simulink model "E"  (R2024a)
settings: Solver=VariableStepAuto  StartTime=0.0  StopTime=10*10^-6  RelTol=1e-3
undefined symbols (not defined in the file): c1, c3, rxDpIndex
libraries: commblkcod2 x64, commofdm x64, commdigbbndam3 x64, commsink2 x1, commseqgen3 x1
(part 3 of 3)

== system E/Subsystem1/MCS13 WiFi Demodulator25 ==
  In1 : Inport
  BCH Decoder1 : commblkcod2/BCH Decoder  n=47040  k=39200  specShortening=off  shortenedK=5  specGenPoly=off  genPoly='X^10 + X^8 + X^5 + X^4 + X^2 + X + 1'  specPrimPoly=off  prPoly='X^4 + X + 1'  specDisableGenCheck=off  specPuncture=off  punctVec=[ones(8,1); zeros(2,1)]  specErasurePort=off  showNumErr=off
  OFDM Demodulator1 : commofdm/OFDM Demodulator  StatePerturbationForJacobian=1.0e-05  FFTLength=4096  NumGuardBandCarriers=[88; 88]  RemoveDCCarrier=off  PilotOutputPort=off  PilotCarrierIndices=[35;60;85;110;135;160;185;210;235;260;285;310;335;360;385;410;435;460;485;510;535;560;585;610;635;660;685;710;735;760;785;810;835;860;885;910;935;960;985;1010;1035;1060;1085;1110;1135;1160;1185;1210;1235;1260;1285;1310;1335;1360;1385;1410;1435;1460;1485;1510;1535;1560;1585;1610;1635;1660;1685;1710;1735;1760;1785;1810;1835;1860;1885;1910;1935;1960;1985;2010;2035]  CyclicPrefixLength=0  OversamplingFactor=1  NumSymbols=1  NumReceiveAntennas=1  SimulateUsing=Interpreted execution
  Rectangular QAM Demodulator Baseband1 : commdigbbndam3/Rectangular QAM Demodulator Baseband  M=4096  OutType=Bit  DecType=Hard decision  VarSource=Dialog  Variance=1  Dec=Gray  Mapping=[0:15]  PowType=Min. distance between symbols  MinDist=2  AvgPow=1  PeakPow=1  Ph=0  outDtype1=Inherit via internal rule  outDtype2=Inherit via internal rule  derotateFactorWordLen=16  derotateFactorDataTypeStr=Inherit: Same word length as input  derotateFactorLastDataTypeStr=Inherit: Same word length as input  denormFactorWordLen=16  denormFactorDataTypeStr=Inherit: Same word length as input  denormFactorLastDataTypeStr=Inherit: Same word length as input  prodOutWordLen=32  prodOutOverflowMode=Wrap  prodOutRoundingMode=Floor  prodOutOvFlMode=off  prodOutOvFlModeLastStrValue=off  sumWordLen=32
      settings: LibrarySourceBlock=|
      | commhdldigbbndam/Rectangular QAM
      | Demodulator
      | Baseband
  Out1 : Outport
  wires:
  BCH Decoder1/1 -> Out1/1
  OFDM Demodulator1/1 -> Rectangular QAM Demodulator Baseband1/1
  In1/1 -> OFDM Demodulator1/1
  Rectangular QAM Demodulator Baseband1/1 -> BCH Decoder1/1

== system E/Subsystem1/MCS13 WiFi Demodulator26 ==
  In1 : Inport
  BCH Decoder1 : commblkcod2/BCH Decoder  n=47040  k=39200  specShortening=off  shortenedK=5  specGenPoly=off  genPoly='X^10 + X^8 + X^5 + X^4 + X^2 + X + 1'  specPrimPoly=off  prPoly='X^4 + X + 1'  specDisableGenCheck=off  specPuncture=off  punctVec=[ones(8,1); zeros(2,1)]  specErasurePort=off  showNumErr=off
  OFDM Demodulator1 : commofdm/OFDM Demodulator  StatePerturbationForJacobian=1.0e-05  FFTLength=4096  NumGuardBandCarriers=[88; 88]  RemoveDCCarrier=off  PilotOutputPort=off  PilotCarrierIndices=[35;60;85;110;135;160;185;210;235;260;285;310;335;360;385;410;435;460;485;510;535;560;585;610;635;660;685;710;735;760;785;810;835;860;885;910;935;960;985;1010;1035;1060;1085;1110;1135;1160;1185;1210;1235;1260;1285;1310;1335;1360;1385;1410;1435;1460;1485;1510;1535;1560;1585;1610;1635;1660;1685;1710;1735;1760;1785;1810;1835;1860;1885;1910;1935;1960;1985;2010;2035]  CyclicPrefixLength=0  OversamplingFactor=1  NumSymbols=1  NumReceiveAntennas=1  SimulateUsing=Interpreted execution
  Rectangular QAM Demodulator Baseband1 : commdigbbndam3/Rectangular QAM Demodulator Baseband  M=4096  OutType=Bit  DecType=Hard decision  VarSource=Dialog  Variance=1  Dec=Gray  Mapping=[0:15]  PowType=Min. distance between symbols  MinDist=2  AvgPow=1  PeakPow=1  Ph=0  outDtype1=Inherit via internal rule  outDtype2=Inherit via internal rule  derotateFactorWordLen=16  derotateFactorDataTypeStr=Inherit: Same word length as input  derotateFactorLastDataTypeStr=Inherit: Same word length as input  denormFactorWordLen=16  denormFactorDataTypeStr=Inherit: Same word length as input  denormFactorLastDataTypeStr=Inherit: Same word length as input  prodOutWordLen=32  prodOutOverflowMode=Wrap  prodOutRoundingMode=Floor  prodOutOvFlMode=off  prodOutOvFlModeLastStrValue=off  sumWordLen=32
      settings: LibrarySourceBlock=|
      | commhdldigbbndam/Rectangular QAM
      | Demodulator
      | Baseband
  Out1 : Outport
  wires:
  BCH Decoder1/1 -> Out1/1
  OFDM Demodulator1/1 -> Rectangular QAM Demodulator Baseband1/1
  In1/1 -> OFDM Demodulator1/1
  Rectangular QAM Demodulator Baseband1/1 -> BCH Decoder1/1

== system E/Subsystem1/MCS13 WiFi Demodulator27 ==
  In1 : Inport
  BCH Decoder1 : commblkcod2/BCH Decoder  n=47040  k=39200  specShortening=off  shortenedK=5  specGenPoly=off  genPoly='X^10 + X^8 + X^5 + X^4 + X^2 + X + 1'  specPrimPoly=off  prPoly='X^4 + X + 1'  specDisableGenCheck=off  specPuncture=off  punctVec=[ones(8,1); zeros(2,1)]  specErasurePort=off  showNumErr=off
  OFDM Demodulator1 : commofdm/OFDM Demodulator  StatePerturbationForJacobian=1.0e-05  FFTLength=4096  NumGuardBandCarriers=[88; 88]  RemoveDCCarrier=off  PilotOutputPort=off  PilotCarrierIndices=[35;60;85;110;135;160;185;210;235;260;285;310;335;360;385;410;435;460;485;510;535;560;585;610;635;660;685;710;735;760;785;810;835;860;885;910;935;960;985;1010;1035;1060;1085;1110;1135;1160;1185;1210;1235;1260;1285;1310;1335;1360;1385;1410;1435;1460;1485;1510;1535;1560;1585;1610;1635;1660;1685;1710;1735;1760;1785;1810;1835;1860;1885;1910;1935;1960;1985;2010;2035]  CyclicPrefixLength=0  OversamplingFactor=1  NumSymbols=1  NumReceiveAntennas=1  SimulateUsing=Interpreted execution
  Rectangular QAM Demodulator Baseband1 : commdigbbndam3/Rectangular QAM Demodulator Baseband  M=4096  OutType=Bit  DecType=Hard decision  VarSource=Dialog  Variance=1  Dec=Gray  Mapping=[0:15]  PowType=Min. distance between symbols  MinDist=2  AvgPow=1  PeakPow=1  Ph=0  outDtype1=Inherit via internal rule  outDtype2=Inherit via internal rule  derotateFactorWordLen=16  derotateFactorDataTypeStr=Inherit: Same word length as input  derotateFactorLastDataTypeStr=Inherit: Same word length as input  denormFactorWordLen=16  denormFactorDataTypeStr=Inherit: Same word length as input  denormFactorLastDataTypeStr=Inherit: Same word length as input  prodOutWordLen=32  prodOutOverflowMode=Wrap  prodOutRoundingMode=Floor  prodOutOvFlMode=off  prodOutOvFlModeLastStrValue=off  sumWordLen=32
      settings: LibrarySourceBlock=|
      | commhdldigbbndam/Rectangular QAM
      | Demodulator
      | Baseband
  Out1 : Outport
  wires:
  BCH Decoder1/1 -> Out1/1
  OFDM Demodulator1/1 -> Rectangular QAM Demodulator Baseband1/1
  In1/1 -> OFDM Demodulator1/1
  Rectangular QAM Demodulator Baseband1/1 -> BCH Decoder1/1

== system E/Subsystem1/MCS13 WiFi Demodulator28 ==
  In1 : Inport
  BCH Decoder1 : commblkcod2/BCH Decoder  n=47040  k=39200  specShortening=off  shortenedK=5  specGenPoly=off  genPoly='X^10 + X^8 + X^5 + X^4 + X^2 + X + 1'  specPrimPoly=off  prPoly='X^4 + X + 1'  specDisableGenCheck=off  specPuncture=off  punctVec=[ones(8,1); zeros(2,1)]  specErasurePort=off  showNumErr=off
  OFDM Demodulator1 : commofdm/OFDM Demodulator  StatePerturbationForJacobian=1.0e-05  FFTLength=4096  NumGuardBandCarriers=[88; 88]  RemoveDCCarrier=off  PilotOutputPort=off  PilotCarrierIndices=[35;60;85;110;135;160;185;210;235;260;285;310;335;360;385;410;435;460;485;510;535;560;585;610;635;660;685;710;735;760;785;810;835;860;885;910;935;960;985;1010;1035;1060;1085;1110;1135;1160;1185;1210;1235;1260;1285;1310;1335;1360;1385;1410;1435;1460;1485;1510;1535;1560;1585;1610;1635;1660;1685;1710;1735;1760;1785;1810;1835;1860;1885;1910;1935;1960;1985;2010;2035]  CyclicPrefixLength=0  OversamplingFactor=1  NumSymbols=1  NumReceiveAntennas=1  SimulateUsing=Interpreted execution
  Rectangular QAM Demodulator Baseband1 : commdigbbndam3/Rectangular QAM Demodulator Baseband  M=4096  OutType=Bit  DecType=Hard decision  VarSource=Dialog  Variance=1  Dec=Gray  Mapping=[0:15]  PowType=Min. distance between symbols  MinDist=2  AvgPow=1  PeakPow=1  Ph=0  outDtype1=Inherit via internal rule  outDtype2=Inherit via internal rule  derotateFactorWordLen=16  derotateFactorDataTypeStr=Inherit: Same word length as input  derotateFactorLastDataTypeStr=Inherit: Same word length as input  denormFactorWordLen=16  denormFactorDataTypeStr=Inherit: Same word length as input  denormFactorLastDataTypeStr=Inherit: Same word length as input  prodOutWordLen=32  prodOutOverflowMode=Wrap  prodOutRoundingMode=Floor  prodOutOvFlMode=off  prodOutOvFlModeLastStrValue=off  sumWordLen=32
      settings: LibrarySourceBlock=|
      | commhdldigbbndam/Rectangular QAM
      | Demodulator
      | Baseband
  Out1 : Outport
  wires:
  BCH Decoder1/1 -> Out1/1
  OFDM Demodulator1/1 -> Rectangular QAM Demodulator Baseband1/1
  In1/1 -> OFDM Demodulator1/1
  Rectangular QAM Demodulator Baseband1/1 -> BCH Decoder1/1

== system E/Subsystem1/MCS13 WiFi Demodulator29 ==
  In1 : Inport
  BCH Decoder1 : commblkcod2/BCH Decoder  n=47040  k=39200  specShortening=off  shortenedK=5  specGenPoly=off  genPoly='X^10 + X^8 + X^5 + X^4 + X^2 + X + 1'  specPrimPoly=off  prPoly='X^4 + X + 1'  specDisableGenCheck=off  specPuncture=off  punctVec=[ones(8,1); zeros(2,1)]  specErasurePort=off  showNumErr=off
  OFDM Demodulator1 : commofdm/OFDM Demodulator  StatePerturbationForJacobian=1.0e-05  FFTLength=4096  NumGuardBandCarriers=[88; 88]  RemoveDCCarrier=off  PilotOutputPort=off  PilotCarrierIndices=[35;60;85;110;135;160;185;210;235;260;285;310;335;360;385;410;435;460;485;510;535;560;585;610;635;660;685;710;735;760;785;810;835;860;885;910;935;960;985;1010;1035;1060;1085;1110;1135;1160;1185;1210;1235;1260;1285;1310;1335;1360;1385;1410;1435;1460;1485;1510;1535;1560;1585;1610;1635;1660;1685;1710;1735;1760;1785;1810;1835;1860;1885;1910;1935;1960;1985;2010;2035]  CyclicPrefixLength=0  OversamplingFactor=1  NumSymbols=1  NumReceiveAntennas=1  SimulateUsing=Interpreted execution
  Rectangular QAM Demodulator Baseband1 : commdigbbndam3/Rectangular QAM Demodulator Baseband  M=4096  OutType=Bit  DecType=Hard decision  VarSource=Dialog  Variance=1  Dec=Gray  Mapping=[0:15]  PowType=Min. distance between symbols  MinDist=2  AvgPow=1  PeakPow=1  Ph=0  outDtype1=Inherit via internal rule  outDtype2=Inherit via internal rule  derotateFactorWordLen=16  derotateFactorDataTypeStr=Inherit: Same word length as input  derotateFactorLastDataTypeStr=Inherit: Same word length as input  denormFactorWordLen=16  denormFactorDataTypeStr=Inherit: Same word length as input  denormFactorLastDataTypeStr=Inherit: Same word length as input  prodOutWordLen=32  prodOutOverflowMode=Wrap  prodOutRoundingMode=Floor  prodOutOvFlMode=off  prodOutOvFlModeLastStrValue=off  sumWordLen=32
      settings: LibrarySourceBlock=|
      | commhdldigbbndam/Rectangular QAM
      | Demodulator
      | Baseband
  Out1 : Outport
  wires:
  BCH Decoder1/1 -> Out1/1
  OFDM Demodulator1/1 -> Rectangular QAM Demodulator Baseband1/1
  In1/1 -> OFDM Demodulator1/1
  Rectangular QAM Demodulator Baseband1/1 -> BCH Decoder1/1

== system E/Subsystem1/MCS13 WiFi Demodulator3 ==
  In1 : Inport
  BCH Decoder1 : commblkcod2/BCH Decoder  n=47040  k=39200  specShortening=off  shortenedK=5  specGenPoly=off  genPoly='X^10 + X^8 + X^5 + X^4 + X^2 + X + 1'  specPrimPoly=off  prPoly='X^4 + X + 1'  specDisableGenCheck=off  specPuncture=off  punctVec=[ones(8,1); zeros(2,1)]  specErasurePort=off  showNumErr=off
  OFDM Demodulator1 : commofdm/OFDM Demodulator  StatePerturbationForJacobian=1.0e-05  FFTLength=4096  NumGuardBandCarriers=[88; 88]  RemoveDCCarrier=off  PilotOutputPort=off  PilotCarrierIndices=[35;60;85;110;135;160;185;210;235;260;285;310;335;360;385;410;435;460;485;510;535;560;585;610;635;660;685;710;735;760;785;810;835;860;885;910;935;960;985;1010;1035;1060;1085;1110;1135;1160;1185;1210;1235;1260;1285;1310;1335;1360;1385;1410;1435;1460;1485;1510;1535;1560;1585;1610;1635;1660;1685;1710;1735;1760;1785;1810;1835;1860;1885;1910;1935;1960;1985;2010;2035]  CyclicPrefixLength=0  OversamplingFactor=1  NumSymbols=1  NumReceiveAntennas=1  SimulateUsing=Interpreted execution
  Rectangular QAM Demodulator Baseband1 : commdigbbndam3/Rectangular QAM Demodulator Baseband  M=4096  OutType=Bit  DecType=Hard decision  VarSource=Dialog  Variance=1  Dec=Gray  Mapping=[0:15]  PowType=Min. distance between symbols  MinDist=2  AvgPow=1  PeakPow=1  Ph=0  outDtype1=Inherit via internal rule  outDtype2=Inherit via internal rule  derotateFactorWordLen=16  derotateFactorDataTypeStr=Inherit: Same word length as input  derotateFactorLastDataTypeStr=Inherit: Same word length as input  denormFactorWordLen=16  denormFactorDataTypeStr=Inherit: Same word length as input  denormFactorLastDataTypeStr=Inherit: Same word length as input  prodOutWordLen=32  prodOutOverflowMode=Wrap  prodOutRoundingMode=Floor  prodOutOvFlMode=off  prodOutOvFlModeLastStrValue=off  sumWordLen=32
      settings: LibrarySourceBlock=|
      | commhdldigbbndam/Rectangular QAM
      | Demodulator
      | Baseband
  Out1 : Outport
  wires:
  BCH Decoder1/1 -> Out1/1
  OFDM Demodulator1/1 -> Rectangular QAM Demodulator Baseband1/1
  In1/1 -> OFDM Demodulator1/1
  Rectangular QAM Demodulator Baseband1/1 -> BCH Decoder1/1

== system E/Subsystem1/MCS13 WiFi Demodulator30 ==
  In1 : Inport
  BCH Decoder1 : commblkcod2/BCH Decoder  n=47040  k=39200  specShortening=off  shortenedK=5  specGenPoly=off  genPoly='X^10 + X^8 + X^5 + X^4 + X^2 + X + 1'  specPrimPoly=off  prPoly='X^4 + X + 1'  specDisableGenCheck=off  specPuncture=off  punctVec=[ones(8,1); zeros(2,1)]  specErasurePort=off  showNumErr=off
  OFDM Demodulator1 : commofdm/OFDM Demodulator  StatePerturbationForJacobian=1.0e-05  FFTLength=4096  NumGuardBandCarriers=[88; 88]  RemoveDCCarrier=off  PilotOutputPort=off  PilotCarrierIndices=[35;60;85;110;135;160;185;210;235;260;285;310;335;360;385;410;435;460;485;510;535;560;585;610;635;660;685;710;735;760;785;810;835;860;885;910;935;960;985;1010;1035;1060;1085;1110;1135;1160;1185;1210;1235;1260;1285;1310;1335;1360;1385;1410;1435;1460;1485;1510;1535;1560;1585;1610;1635;1660;1685;1710;1735;1760;1785;1810;1835;1860;1885;1910;1935;1960;1985;2010;2035]  CyclicPrefixLength=0  OversamplingFactor=1  NumSymbols=1  NumReceiveAntennas=1  SimulateUsing=Interpreted execution
  Rectangular QAM Demodulator Baseband1 : commdigbbndam3/Rectangular QAM Demodulator Baseband  M=4096  OutType=Bit  DecType=Hard decision  VarSource=Dialog  Variance=1  Dec=Gray  Mapping=[0:15]  PowType=Min. distance between symbols  MinDist=2  AvgPow=1  PeakPow=1  Ph=0  outDtype1=Inherit via internal rule  outDtype2=Inherit via internal rule  derotateFactorWordLen=16  derotateFactorDataTypeStr=Inherit: Same word length as input  derotateFactorLastDataTypeStr=Inherit: Same word length as input  denormFactorWordLen=16  denormFactorDataTypeStr=Inherit: Same word length as input  denormFactorLastDataTypeStr=Inherit: Same word length as input  prodOutWordLen=32  prodOutOverflowMode=Wrap  prodOutRoundingMode=Floor  prodOutOvFlMode=off  prodOutOvFlModeLastStrValue=off  sumWordLen=32
      settings: LibrarySourceBlock=|
      | commhdldigbbndam/Rectangular QAM
      | Demodulator
      | Baseband
  Out1 : Outport
  wires:
  BCH Decoder1/1 -> Out1/1
  OFDM Demodulator1/1 -> Rectangular QAM Demodulator Baseband1/1
  In1/1 -> OFDM Demodulator1/1
  Rectangular QAM Demodulator Baseband1/1 -> BCH Decoder1/1

== system E/Subsystem1/MCS13 WiFi Demodulator31 ==
  In1 : Inport
  BCH Decoder1 : commblkcod2/BCH Decoder  n=47040  k=39200  specShortening=off  shortenedK=5  specGenPoly=off  genPoly='X^10 + X^8 + X^5 + X^4 + X^2 + X + 1'  specPrimPoly=off  prPoly='X^4 + X + 1'  specDisableGenCheck=off  specPuncture=off  punctVec=[ones(8,1); zeros(2,1)]  specErasurePort=off  showNumErr=off
  OFDM Demodulator1 : commofdm/OFDM Demodulator  StatePerturbationForJacobian=1.0e-05  FFTLength=4096  NumGuardBandCarriers=[88; 88]  RemoveDCCarrier=off  PilotOutputPort=off  PilotCarrierIndices=[35;60;85;110;135;160;185;210;235;260;285;310;335;360;385;410;435;460;485;510;535;560;585;610;635;660;685;710;735;760;785;810;835;860;885;910;935;960;985;1010;1035;1060;1085;1110;1135;1160;1185;1210;1235;1260;1285;1310;1335;1360;1385;1410;1435;1460;1485;1510;1535;1560;1585;1610;1635;1660;1685;1710;1735;1760;1785;1810;1835;1860;1885;1910;1935;1960;1985;2010;2035]  CyclicPrefixLength=0  OversamplingFactor=1  NumSymbols=1  NumReceiveAntennas=1  SimulateUsing=Interpreted execution
  Rectangular QAM Demodulator Baseband1 : commdigbbndam3/Rectangular QAM Demodulator Baseband  M=4096  OutType=Bit  DecType=Hard decision  VarSource=Dialog  Variance=1  Dec=Gray  Mapping=[0:15]  PowType=Min. distance between symbols  MinDist=2  AvgPow=1  PeakPow=1  Ph=0  outDtype1=Inherit via internal rule  outDtype2=Inherit via internal rule  derotateFactorWordLen=16  derotateFactorDataTypeStr=Inherit: Same word length as input  derotateFactorLastDataTypeStr=Inherit: Same word length as input  denormFactorWordLen=16  denormFactorDataTypeStr=Inherit: Same word length as input  denormFactorLastDataTypeStr=Inherit: Same word length as input  prodOutWordLen=32  prodOutOverflowMode=Wrap  prodOutRoundingMode=Floor  prodOutOvFlMode=off  prodOutOvFlModeLastStrValue=off  sumWordLen=32
      settings: LibrarySourceBlock=|
      | commhdldigbbndam/Rectangular QAM
      | Demodulator
      | Baseband
  Out1 : Outport
  wires:
  BCH Decoder1/1 -> Out1/1
  OFDM Demodulator1/1 -> Rectangular QAM Demodulator Baseband1/1
  In1/1 -> OFDM Demodulator1/1
  Rectangular QAM Demodulator Baseband1/1 -> BCH Decoder1/1

== system E/Subsystem1/MCS13 WiFi Demodulator32 ==
  In1 : Inport
  BCH Decoder1 : commblkcod2/BCH Decoder  n=47040  k=39200  specShortening=off  shortenedK=5  specGenPoly=off  genPoly='X^10 + X^8 + X^5 + X^4 + X^2 + X + 1'  specPrimPoly=off  prPoly='X^4 + X + 1'  specDisableGenCheck=off  specPuncture=off  punctVec=[ones(8,1); zeros(2,1)]  specErasurePort=off  showNumErr=off
  OFDM Demodulator1 : commofdm/OFDM Demodulator  StatePerturbationForJacobian=1.0e-05  FFTLength=4096  NumGuardBandCarriers=[88; 88]  RemoveDCCarrier=off  PilotOutputPort=off  PilotCarrierIndices=[35;60;85;110;135;160;185;210;235;260;285;310;335;360;385;410;435;460;485;510;535;560;585;610;635;660;685;710;735;760;785;810;835;860;885;910;935;960;985;1010;1035;1060;1085;1110;1135;1160;1185;1210;1235;1260;1285;1310;1335;1360;1385;1410;1435;1460;1485;1510;1535;1560;1585;1610;1635;1660;1685;1710;1735;1760;1785;1810;1835;1860;1885;1910;1935;1960;1985;2010;2035]  CyclicPrefixLength=0  OversamplingFactor=1  NumSymbols=1  NumReceiveAntennas=1  SimulateUsing=Interpreted execution
  Rectangular QAM Demodulator Baseband1 : commdigbbndam3/Rectangular QAM Demodulator Baseband  M=4096  OutType=Bit  DecType=Hard decision  VarSource=Dialog  Variance=1  Dec=Gray  Mapping=[0:15]  PowType=Min. distance between symbols  MinDist=2  AvgPow=1  PeakPow=1  Ph=0  outDtype1=Inherit via internal rule  outDtype2=Inherit via internal rule  derotateFactorWordLen=16  derotateFactorDataTypeStr=Inherit: Same word length as input  derotateFactorLastDataTypeStr=Inherit: Same word length as input  denormFactorWordLen=16  denormFactorDataTypeStr=Inherit: Same word length as input  denormFactorLastDataTypeStr=Inherit: Same word length as input  prodOutWordLen=32  prodOutOverflowMode=Wrap  prodOutRoundingMode=Floor  prodOutOvFlMode=off  prodOutOvFlModeLastStrValue=off  sumWordLen=32
      settings: LibrarySourceBlock=|
      | commhdldigbbndam/Rectangular QAM
      | Demodulator
      | Baseband
  Out1 : Outport
  wires:
  BCH Decoder1/1 -> Out1/1
  OFDM Demodulator1/1 -> Rectangular QAM Demodulator Baseband1/1
  In1/1 -> OFDM Demodulator1/1
  Rectangular QAM Demodulator Baseband1/1 -> BCH Decoder1/1

== system E/Subsystem1/MCS13 WiFi Demodulator4 ==
  In1 : Inport
  BCH Decoder1 : commblkcod2/BCH Decoder  n=47040  k=39200  specShortening=off  shortenedK=5  specGenPoly=off  genPoly='X^10 + X^8 + X^5 + X^4 + X^2 + X + 1'  specPrimPoly=off  prPoly='X^4 + X + 1'  specDisableGenCheck=off  specPuncture=off  punctVec=[ones(8,1); zeros(2,1)]  specErasurePort=off  showNumErr=off
  OFDM Demodulator1 : commofdm/OFDM Demodulator  StatePerturbationForJacobian=1.0e-05  FFTLength=4096  NumGuardBandCarriers=[88; 88]  RemoveDCCarrier=off  PilotOutputPort=off  PilotCarrierIndices=[35;60;85;110;135;160;185;210;235;260;285;310;335;360;385;410;435;460;485;510;535;560;585;610;635;660;685;710;735;760;785;810;835;860;885;910;935;960;985;1010;1035;1060;1085;1110;1135;1160;1185;1210;1235;1260;1285;1310;1335;1360;1385;1410;1435;1460;1485;1510;1535;1560;1585;1610;1635;1660;1685;1710;1735;1760;1785;1810;1835;1860;1885;1910;1935;1960;1985;2010;2035]  CyclicPrefixLength=0  OversamplingFactor=1  NumSymbols=1  NumReceiveAntennas=1  SimulateUsing=Interpreted execution
  Rectangular QAM Demodulator Baseband1 : commdigbbndam3/Rectangular QAM Demodulator Baseband  M=4096  OutType=Bit  DecType=Hard decision  VarSource=Dialog  Variance=1  Dec=Gray  Mapping=[0:15]  PowType=Min. distance between symbols  MinDist=2  AvgPow=1  PeakPow=1  Ph=0  outDtype1=Inherit via internal rule  outDtype2=Inherit via internal rule  derotateFactorWordLen=16  derotateFactorDataTypeStr=Inherit: Same word length as input  derotateFactorLastDataTypeStr=Inherit: Same word length as input  denormFactorWordLen=16  denormFactorDataTypeStr=Inherit: Same word length as input  denormFactorLastDataTypeStr=Inherit: Same word length as input  prodOutWordLen=32  prodOutOverflowMode=Wrap  prodOutRoundingMode=Floor  prodOutOvFlMode=off  prodOutOvFlModeLastStrValue=off  sumWordLen=32
      settings: LibrarySourceBlock=|
      | commhdldigbbndam/Rectangular QAM
      | Demodulator
      | Baseband
  Out1 : Outport
  wires:
  BCH Decoder1/1 -> Out1/1
  OFDM Demodulator1/1 -> Rectangular QAM Demodulator Baseband1/1
  In1/1 -> OFDM Demodulator1/1
  Rectangular QAM Demodulator Baseband1/1 -> BCH Decoder1/1

== system E/Subsystem1/MCS13 WiFi Demodulator5 ==
  In1 : Inport
  BCH Decoder1 : commblkcod2/BCH Decoder  n=47040  k=39200  specShortening=off  shortenedK=5  specGenPoly=off  genPoly='X^10 + X^8 + X^5 + X^4 + X^2 + X + 1'  specPrimPoly=off  prPoly='X^4 + X + 1'  specDisableGenCheck=off  specPuncture=off  punctVec=[ones(8,1); zeros(2,1)]  specErasurePort=off  showNumErr=off
  OFDM Demodulator1 : commofdm/OFDM Demodulator  StatePerturbationForJacobian=1.0e-05  FFTLength=4096  NumGuardBandCarriers=[88; 88]  RemoveDCCarrier=off  PilotOutputPort=off  PilotCarrierIndices=[35;60;85;110;135;160;185;210;235;260;285;310;335;360;385;410;435;460;485;510;535;560;585;610;635;660;685;710;735;760;785;810;835;860;885;910;935;960;985;1010;1035;1060;1085;1110;1135;1160;1185;1210;1235;1260;1285;1310;1335;1360;1385;1410;1435;1460;1485;1510;1535;1560;1585;1610;1635;1660;1685;1710;1735;1760;1785;1810;1835;1860;1885;1910;1935;1960;1985;2010;2035]  CyclicPrefixLength=0  OversamplingFactor=1  NumSymbols=1  NumReceiveAntennas=1  SimulateUsing=Interpreted execution
  Rectangular QAM Demodulator Baseband1 : commdigbbndam3/Rectangular QAM Demodulator Baseband  M=4096  OutType=Bit  DecType=Hard decision  VarSource=Dialog  Variance=1  Dec=Gray  Mapping=[0:15]  PowType=Min. distance between symbols  MinDist=2  AvgPow=1  PeakPow=1  Ph=0  outDtype1=Inherit via internal rule  outDtype2=Inherit via internal rule  derotateFactorWordLen=16  derotateFactorDataTypeStr=Inherit: Same word length as input  derotateFactorLastDataTypeStr=Inherit: Same word length as input  denormFactorWordLen=16  denormFactorDataTypeStr=Inherit: Same word length as input  denormFactorLastDataTypeStr=Inherit: Same word length as input  prodOutWordLen=32  prodOutOverflowMode=Wrap  prodOutRoundingMode=Floor  prodOutOvFlMode=off  prodOutOvFlModeLastStrValue=off  sumWordLen=32
      settings: LibrarySourceBlock=|
      | commhdldigbbndam/Rectangular QAM
      | Demodulator
      | Baseband
  Out1 : Outport
  wires:
  BCH Decoder1/1 -> Out1/1
  OFDM Demodulator1/1 -> Rectangular QAM Demodulator Baseband1/1
  In1/1 -> OFDM Demodulator1/1
  Rectangular QAM Demodulator Baseband1/1 -> BCH Decoder1/1

== system E/Subsystem1/MCS13 WiFi Demodulator6 ==
  In1 : Inport
  BCH Decoder1 : commblkcod2/BCH Decoder  n=47040  k=39200  specShortening=off  shortenedK=5  specGenPoly=off  genPoly='X^10 + X^8 + X^5 + X^4 + X^2 + X + 1'  specPrimPoly=off  prPoly='X^4 + X + 1'  specDisableGenCheck=off  specPuncture=off  punctVec=[ones(8,1); zeros(2,1)]  specErasurePort=off  showNumErr=off
  OFDM Demodulator1 : commofdm/OFDM Demodulator  StatePerturbationForJacobian=1.0e-05  FFTLength=4096  NumGuardBandCarriers=[88; 88]  RemoveDCCarrier=off  PilotOutputPort=off  PilotCarrierIndices=[35;60;85;110;135;160;185;210;235;260;285;310;335;360;385;410;435;460;485;510;535;560;585;610;635;660;685;710;735;760;785;810;835;860;885;910;935;960;985;1010;1035;1060;1085;1110;1135;1160;1185;1210;1235;1260;1285;1310;1335;1360;1385;1410;1435;1460;1485;1510;1535;1560;1585;1610;1635;1660;1685;1710;1735;1760;1785;1810;1835;1860;1885;1910;1935;1960;1985;2010;2035]  CyclicPrefixLength=0  OversamplingFactor=1  NumSymbols=1  NumReceiveAntennas=1  SimulateUsing=Interpreted execution
  Rectangular QAM Demodulator Baseband1 : commdigbbndam3/Rectangular QAM Demodulator Baseband  M=4096  OutType=Bit  DecType=Hard decision  VarSource=Dialog  Variance=1  Dec=Gray  Mapping=[0:15]  PowType=Min. distance between symbols  MinDist=2  AvgPow=1  PeakPow=1  Ph=0  outDtype1=Inherit via internal rule  outDtype2=Inherit via internal rule  derotateFactorWordLen=16  derotateFactorDataTypeStr=Inherit: Same word length as input  derotateFactorLastDataTypeStr=Inherit: Same word length as input  denormFactorWordLen=16  denormFactorDataTypeStr=Inherit: Same word length as input  denormFactorLastDataTypeStr=Inherit: Same word length as input  prodOutWordLen=32  prodOutOverflowMode=Wrap  prodOutRoundingMode=Floor  prodOutOvFlMode=off  prodOutOvFlModeLastStrValue=off  sumWordLen=32
      settings: LibrarySourceBlock=|
      | commhdldigbbndam/Rectangular QAM
      | Demodulator
      | Baseband
  Out1 : Outport
  wires:
  BCH Decoder1/1 -> Out1/1
  OFDM Demodulator1/1 -> Rectangular QAM Demodulator Baseband1/1
  In1/1 -> OFDM Demodulator1/1
  Rectangular QAM Demodulator Baseband1/1 -> BCH Decoder1/1

== system E/Subsystem1/MCS13 WiFi Demodulator7 ==
  In1 : Inport
  BCH Decoder1 : commblkcod2/BCH Decoder  n=47040  k=39200  specShortening=off  shortenedK=5  specGenPoly=off  genPoly='X^10 + X^8 + X^5 + X^4 + X^2 + X + 1'  specPrimPoly=off  prPoly='X^4 + X + 1'  specDisableGenCheck=off  specPuncture=off  punctVec=[ones(8,1); zeros(2,1)]  specErasurePort=off  showNumErr=off
  OFDM Demodulator1 : commofdm/OFDM Demodulator  StatePerturbationForJacobian=1.0e-05  FFTLength=4096  NumGuardBandCarriers=[88; 88]  RemoveDCCarrier=off  PilotOutputPort=off  PilotCarrierIndices=[35;60;85;110;135;160;185;210;235;260;285;310;335;360;385;410;435;460;485;510;535;560;585;610;635;660;685;710;735;760;785;810;835;860;885;910;935;960;985;1010;1035;1060;1085;1110;1135;1160;1185;1210;1235;1260;1285;1310;1335;1360;1385;1410;1435;1460;1485;1510;1535;1560;1585;1610;1635;1660;1685;1710;1735;1760;1785;1810;1835;1860;1885;1910;1935;1960;1985;2010;2035]  CyclicPrefixLength=0  OversamplingFactor=1  NumSymbols=1  NumReceiveAntennas=1  SimulateUsing=Interpreted execution
  Rectangular QAM Demodulator Baseband1 : commdigbbndam3/Rectangular QAM Demodulator Baseband  M=4096  OutType=Bit  DecType=Hard decision  VarSource=Dialog  Variance=1  Dec=Gray  Mapping=[0:15]  PowType=Min. distance between symbols  MinDist=2  AvgPow=1  PeakPow=1  Ph=0  outDtype1=Inherit via internal rule  outDtype2=Inherit via internal rule  derotateFactorWordLen=16  derotateFactorDataTypeStr=Inherit: Same word length as input  derotateFactorLastDataTypeStr=Inherit: Same word length as input  denormFactorWordLen=16  denormFactorDataTypeStr=Inherit: Same word length as input  denormFactorLastDataTypeStr=Inherit: Same word length as input  prodOutWordLen=32  prodOutOverflowMode=Wrap  prodOutRoundingMode=Floor  prodOutOvFlMode=off  prodOutOvFlModeLastStrValue=off  sumWordLen=32
      settings: LibrarySourceBlock=|
      | commhdldigbbndam/Rectangular QAM
      | Demodulator
      | Baseband
  Out1 : Outport
  wires:
  BCH Decoder1/1 -> Out1/1
  OFDM Demodulator1/1 -> Rectangular QAM Demodulator Baseband1/1
  In1/1 -> OFDM Demodulator1/1
  Rectangular QAM Demodulator Baseband1/1 -> BCH Decoder1/1

== system E/Subsystem1/MCS13 WiFi Demodulator8 ==
  In1 : Inport
  BCH Decoder1 : commblkcod2/BCH Decoder  n=47040  k=39200  specShortening=off  shortenedK=5  specGenPoly=off  genPoly='X^10 + X^8 + X^5 + X^4 + X^2 + X + 1'  specPrimPoly=off  prPoly='X^4 + X + 1'  specDisableGenCheck=off  specPuncture=off  punctVec=[ones(8,1); zeros(2,1)]  specErasurePort=off  showNumErr=off
  OFDM Demodulator1 : commofdm/OFDM Demodulator  StatePerturbationForJacobian=1.0e-05  FFTLength=4096  NumGuardBandCarriers=[88; 88]  RemoveDCCarrier=off  PilotOutputPort=off  PilotCarrierIndices=[35;60;85;110;135;160;185;210;235;260;285;310;335;360;385;410;435;460;485;510;535;560;585;610;635;660;685;710;735;760;785;810;835;860;885;910;935;960;985;1010;1035;1060;1085;1110;1135;1160;1185;1210;1235;1260;1285;1310;1335;1360;1385;1410;1435;1460;1485;1510;1535;1560;1585;1610;1635;1660;1685;1710;1735;1760;1785;1810;1835;1860;1885;1910;1935;1960;1985;2010;2035]  CyclicPrefixLength=0  OversamplingFactor=1  NumSymbols=1  NumReceiveAntennas=1  SimulateUsing=Interpreted execution
  Rectangular QAM Demodulator Baseband1 : commdigbbndam3/Rectangular QAM Demodulator Baseband  M=4096  OutType=Bit  DecType=Hard decision  VarSource=Dialog  Variance=1  Dec=Gray  Mapping=[0:15]  PowType=Min. distance between symbols  MinDist=2  AvgPow=1  PeakPow=1  Ph=0  outDtype1=Inherit via internal rule  outDtype2=Inherit via internal rule  derotateFactorWordLen=16  derotateFactorDataTypeStr=Inherit: Same word length as input  derotateFactorLastDataTypeStr=Inherit: Same word length as input  denormFactorWordLen=16  denormFactorDataTypeStr=Inherit: Same word length as input  denormFactorLastDataTypeStr=Inherit: Same word length as input  prodOutWordLen=32  prodOutOverflowMode=Wrap  prodOutRoundingMode=Floor  prodOutOvFlMode=off  prodOutOvFlModeLastStrValue=off  sumWordLen=32
      settings: LibrarySourceBlock=|
      | commhdldigbbndam/Rectangular QAM
      | Demodulator
      | Baseband
  Out1 : Outport
  wires:
  BCH Decoder1/1 -> Out1/1
  OFDM Demodulator1/1 -> Rectangular QAM Demodulator Baseband1/1
  In1/1 -> OFDM Demodulator1/1
  Rectangular QAM Demodulator Baseband1/1 -> BCH Decoder1/1

== system E/Subsystem1/MCS13 WiFi Demodulator9 ==
  In1 : Inport
  BCH Decoder1 : commblkcod2/BCH Decoder  n=47040  k=39200  specShortening=off  shortenedK=5  specGenPoly=off  genPoly='X^10 + X^8 + X^5 + X^4 + X^2 + X + 1'  specPrimPoly=off  prPoly='X^4 + X + 1'  specDisableGenCheck=off  specPuncture=off  punctVec=[ones(8,1); zeros(2,1)]  specErasurePort=off  showNumErr=off
  OFDM Demodulator1 : commofdm/OFDM Demodulator  StatePerturbationForJacobian=1.0e-05  FFTLength=4096  NumGuardBandCarriers=[88; 88]  RemoveDCCarrier=off  PilotOutputPort=off  PilotCarrierIndices=[35;60;85;110;135;160;185;210;235;260;285;310;335;360;385;410;435;460;485;510;535;560;585;610;635;660;685;710;735;760;785;810;835;860;885;910;935;960;985;1010;1035;1060;1085;1110;1135;1160;1185;1210;1235;1260;1285;1310;1335;1360;1385;1410;1435;1460;1485;1510;1535;1560;1585;1610;1635;1660;1685;1710;1735;1760;1785;1810;1835;1860;1885;1910;1935;1960;1985;2010;2035]  CyclicPrefixLength=0  OversamplingFactor=1  NumSymbols=1  NumReceiveAntennas=1  SimulateUsing=Interpreted execution
  Rectangular QAM Demodulator Baseband1 : commdigbbndam3/Rectangular QAM Demodulator Baseband  M=4096  OutType=Bit  DecType=Hard decision  VarSource=Dialog  Variance=1  Dec=Gray  Mapping=[0:15]  PowType=Min. distance between symbols  MinDist=2  AvgPow=1  PeakPow=1  Ph=0  outDtype1=Inherit via internal rule  outDtype2=Inherit via internal rule  derotateFactorWordLen=16  derotateFactorDataTypeStr=Inherit: Same word length as input  derotateFactorLastDataTypeStr=Inherit: Same word length as input  denormFactorWordLen=16  denormFactorDataTypeStr=Inherit: Same word length as input  denormFactorLastDataTypeStr=Inherit: Same word length as input  prodOutWordLen=32  prodOutOverflowMode=Wrap  prodOutRoundingMode=Floor  prodOutOvFlMode=off  prodOutOvFlModeLastStrValue=off  sumWordLen=32
      settings: LibrarySourceBlock=|
      | commhdldigbbndam/Rectangular QAM
      | Demodulator
      | Baseband
  Out1 : Outport
  wires:
  BCH Decoder1/1 -> Out1/1
  OFDM Demodulator1/1 -> Rectangular QAM Demodulator Baseband1/1
  In1/1 -> OFDM Demodulator1/1
  Rectangular QAM Demodulator Baseband1/1 -> BCH Decoder1/1

== matlab function E/     ==
  data: u input; y output; ss input; s output
function [y, s] = fcn(u, ss)

        % Aggregated polarization
        TempAggregatedPolarization = reshape(u', 1, []);
        TAPRowClone = repmat(TempAggregatedPolarization, 32, 1);
        assignin('base', 'PA', TAPRowClone);

        % Aggregated streams
        TempAggregatedProcessedInput = reshape(ss, 1, 131072);
        TAPIRowClone = repmat(TempAggregatedProcessedInput, 32, 1);
        
y = TAPRowClone;
s = TAPIRowClone;

== matlab function E/  ==
  data: u input; y output; ss input; c1 parameter; c3 parameter
function y = fcn(u, ss, c1, c3)
        
        Walsh = [
            1	1	1	1	1	1	1	1	1	1	1	1	1	1	1	1	1	1	1	1	1	1	1	1	1	1	1	1	1	1	1	1;
																															    
            1	-1	1	-1	1	-1	1	-1	1	-1	1	-1	1	-1	1	-1	1	-1	1	-1	1	-1	1	-1	1	-1	1	-1	1	-1	1	-1;
																															            
            1	1	-1	-1	1	1	-1	-1	1	1	-1	-1	1	1	-1	-1	1	1	-1	-1	1	1	-1	-1	1	1	-1	-1	1	1	-1	-1;
																															            
            1	-1	-1	1	1	-1	-1	1	1	-1	-1	1	1	-1	-1	1	1	-1	-1	1	1	-1	-1	1	1	-1	-1	1	1	-1	-1	1;
																															            
            1	1	1	1	-1	-1	-1	-1	1	1	1	1	-1	-1	-1	-1	1	1	1	1	-1	-1	-1	-1	1	1	1	1	-1	-1	-1	-1;
																															            
            1	-1	1	-1	-1	1	-1	1	1	-1	1	-1	-1	1	-1	1	1	-1	1	-1	-1	1	-1	1	1	-1	1	-1	-1	1	-1	1;
																															            
            1	1	-1	-1	-1	-1	1	1	1	1	-1	-1	-1	-1	1	1	1	1	-1	-1	-1	-1	1	1	1	1	-1	-1	-1	-1	1	1;
																															            
            1	-1	-1	1	-1	1	1	-1	1	-1	-1	1	-1	1	1	-1	1	-1	-1	1	-1	1	1	-1	1	-1	-1	1	-1	1	1	-1;
																															            
            1	1	1	1	1	1	1	1	-1	-1	-1	-1	-1	-1	-1	-1	1	1	1	1	1	1	1	1	-1	-1	-1	-1	-1	-1	-1	-1;
																															            
            1	-1	1	-1	1	-1	1	-1	-1	1	-1	1	-1	1	-1	1	1	-1	1	-1	1	-1	1	-1	-1	1	-1	1	-1	1	-1	1;
																															            
            1	1	-1	-1	1	1	-1	-1	-1	-1	1	1	-1	-1	1	1	1	1	-1	-1	1	1	-1	-1	-1	-1	1	1	-1	-1	1	1;
																															            
            1	-1	-1	1	1	-1	-1	1	-1	1	1	-1	-1	1	1	-1	1	-1	-1	1	1	-1	-1	1	-1	1	1	-1	-1	1	1	-1;
																															            
            1	1	1	1	-1	-1	-1	-1	-1	-1	-1	-1	1	1	1	1	1	1	1	1	-1	-1	-1	-1	-1	-1	-1	-1	1	1	1	1;
																															            
            1	-1	1	-1	-1	1	-1	1	-1	1	-1	1	1	-1	1	-1	1	-1	1	-1	-1	1	-1	1	-1	1	-1	1	1	-1	1	-1;
																															            
            1	1	-1	-1	-1	-1	1	1	-1	-1	1	1	1	1	-1	-1	1	1	-1	-1	-1	-1	1	1	-1	-1	1	1	1	1	-1	-1;
																															            
            1	-1	-1	1	-1	1	1	-1	-1	1	1	-1	1	-1	-1	1	1	-1	-1	1	-1	1	1	-1	-1	1	1	-1	1	-1	-1	1;
																															            
            1	1	1	1	1	1	1	1	1	1	1	1	1	1	1	1	-1	-1	-1	-1	-1	-1	-1	-1	-1	-1	-1	-1	-1	-1	-1	-1;
																															            
            1	-1	1	-1	1	-1	1	-1	1	-1	1	-1	1	-1	1	-1	-1	1	-1	1	-1	1	-1	1	-1	1	-1	1	-1	1	-1	1;
																															            
            1	1	-1	-1	1	1	-1	-1	1	1	-1	-1	1	1	-1	-1	-1	-1	1	1	-1	-1	1	1	-1	-1	1	1	-1	-1	1	1;
																															            
            1	-1	-1	1	1	-1	-1	1	1	-1	-1	1	1	-1	-1	1	-1	1	1	-1	-1	1	1	-1	-1	1	1	-1	-1	1	1	-1;
																															            
            1	1	1	1	-1	-1	-1	-1	1	1	1	1	-1	-1	-1	-1	-1	-1	-1	-1	1	1	1	1	-1	-1	-1	-1	1	1	1	1;
																															            
            1	-1	1	-1	-1	1	-1	1	1	-1	1	-1	-1	1	-1	1	-1	1	-1	1	1	-1	1	-1	-1	1	-1	1	1	-1	1	-1;
																															            
            1	1	-1	-1	-1	-1	1	1	1	1	-1	-1	-1	-1	1	1	-1	-1	1	1	1	1	-1	-1	-1	-1	1	1	1	1	-1	-1;
																															            
            1	-1	-1	1	-1	1	1	-1	1	-1	-1	1	-1	1	1	-1	-1	1	1	-1	1	-1	-1	1	-1	1	1	-1	1	-1	-1	1;
																															            
            1	1	1	1	1	1	1	1	-1	-1	-1	-1	-1	-1	-1	-1	-1	-1	-1	-1	-1	-1	-1	-1	1	1	1	1	1	1	1	1;
																															            
            1	-1	1	-1	1	-1	1	-1	-1	1	-1	1	-1	1	-1	1	-1	1	-1	1	-1	1	-1	1	1	-1	1	-1	1	-1	1	-1;
																															            
            1	1	-1	-1	1	1	-1	-1	-1	-1	1	1	-1	-1	1	1	-1	-1	1	1	-1	-1	1	1	1	1	-1	-1	1	1	-1	-1;
																															            
            1	-1	-1	1	1	-1	-1	1	-1	1	1	-1	-1	1	1	-1	-1	1	1	-1	-1	1	1	-1	1	-1	-1	1	1	-1	-1	1;
																															            
            1	1	1	1	-1	-1	-1	-1	-1	-1	-1	-1	1	1	1	1	-1	-1	-1	-1	1	1	1	1	1	1	1	1	-1	-1	-1	-1;
																															            
            1	-1	1	-1	-1	1	-1	1	-1	1	-1	1	1	-1	1	-1	-1	1	-1	1	1	-1	1	-1	1	-1	1	-1	-1	1	-1	1;
																															            
            1	1	-1	-1	-1	-1	1	1	-1	-1	1	1	1	1	-1	-1	-1	-1	1	1	1	1	-1	-1	1	1	-1	-1	-1	-1	1	1;
																															            
            1	-1	-1	1	-1	1	1	-1	-1	1	1	-1	1	-1	-1	1	-1	1	1	-1	1	-1	-1	1	1	-1	-1	1	-1	1	1	-1;
        ];

        Increased_Walsh = Walsh(:, repelem(1:size(Walsh, 2), 16));
        
        Ext_Walsh = repmat(Increased_Walsh, [1, 8]);
        
        % Polarization to be multiplied to Receieved Polarization
        R_matrix = repmat(Ext_Walsh, [1, 32]);
        
        % Multiplication of Polarization and Depolarization
        Result_matrix = u .* R_matrix;
        assignin('base', 'PAD', Result_matrix);
        
        % Sample by sample, Replace 1s with cos, -1s with sin
        % c1 is cos, c3 is sin
        for i = 1:32
            for j = 1:131072

                if Result_matrix(i, j) == 1
                    Result_matrix(i, j) = c1;
                else
                    Result_matrix(i, j) = c3;
                end            

            end
        end

        assignin('base', 'RM1', Result_matrix);
        
        SR_M = rand(32, 32);

        for i = 1:32
            for k = 1:32
                
                start_index = 4096 * (k-1) + 1;
                end_index = start_index + 4095;
                SR_M(i, k) = sum(Result_matrix(i, start_index:end_index))/4096;

            end
        end

        assignin('base', 'SRM', SR_M);

        Result_matrix = repmat(SR_M, [1, 4096]);

        assignin('base', 'RM2', Result_matrix);
       
        % Combine stream with polarization
        Final_matrix = ss .* Result_matrix;
        
        % Pre-matrix to be used for Depolarization matrix
        Depolarized = ss(:, 1:4096);
        
        % Get the depolarized stream matrix: 32*4096
        for i = 1:4096

            col_start = (i-1)*32 + 1;

            col_end = i*32;
            
            Depolarized(:, i) = sum(Final_matrix(:, col_start:col_end), 2);

        end

y = Depolarized;

== matlab function E/  ==
  data: u input; y output; s output
function [y, s] = fcn(u)
    
        Walsh = [
            1	1	1	1	1	1	1	1	1	1	1	1	1	1	1	1	1	1	1	1	1	1	1	1	1	1	1	1	1	1	1	1;
																															    
            1	-1	1	-1	1	-1	1	-1	1	-1	1	-1	1	-1	1	-1	1	-1	1	-1	1	-1	1	-1	1	-1	1	-1	1	-1	1	-1;
																															            
            1	1	-1	-1	1	1	-1	-1	1	1	-1	-1	1	1	-1	-1	1	1	-1	-1	1	1	-1	-1	1	1	-1	-1	1	1	-1	-1;
																															            
            1	-1	-1	1	1	-1	-1	1	1	-1	-1	1	1	-1	-1	1	1	-1	-1	1	1	-1	-1	1	1	-1	-1	1	1	-1	-1	1;
																															            
            1	1	1	1	-1	-1	-1	-1	1	1	1	1	-1	-1	-1	-1	1	1	1	1	-1	-1	-1	-1	1	1	1	1	-1	-1	-1	-1;
																															            
            1	-1	1	-1	-1	1	-1	1	1	-1	1	-1	-1	1	-1	1	1	-1	1	-1	-1	1	-1	1	1	-1	1	-1	-1	1	-1	1;
																															            
            1	1	-1	-1	-1	-1	1	1	1	1	-1	-1	-1	-1	1	1	1	1	-1	-1	-1	-1	1	1	1	1	-1	-1	-1	-1	1	1;
																															            
            1	-1	-1	1	-1	1	1	-1	1	-1	-1	1	-1	1	1	-1	1	-1	-1	1	-1	1	1	-1	1	-1	-1	1	-1	1	1	-1;
																															            
            1	1	1	1	1	1	1	1	-1	-1	-1	-1	-1	-1	-1	-1	1	1	1	1	1	1	1	1	-1	-1	-1	-1	-1	-1	-1	-1;
																															            
            1	-1	1	-1	1	-1	1	-1	-1	1	-1	1	-1	1	-1	1	1	-1	1	-1	1	-1	1	-1	-1	1	-1	1	-1	1	-1	1;
																															            
            1	1	-1	-1	1	1	-1	-1	-1	-1	1	1	-1	-1	1	1	1	1	-1	-1	1	1	-1	-1	-1	-1	1	1	-1	-1	1	1;
																															            
            1	-1	-1	1	1	-1	-1	1	-1	1	1	-1	-1	1	1	-1	1	-1	-1	1	1	-1	-1	1	-1	1	1	-1	-1	1	1	-1;
																															            
            1	1	1	1	-1	-1	-1	-1	-1	-1	-1	-1	1	1	1	1	1	1	1	1	-1	-1	-1	-1	-1	-1	-1	-1	1	1	1	1;
																															            
            1	-1	1	-1	-1	1	-1	1	-1	1	-1	1	1	-1	1	-1	1	-1	1	-1	-1	1	-1	1	-1	1	-1	1	1	-1	1	-1;
																															            
            1	1	-1	-1	-1	-1	1	1	-1	-1	1	1	1	1	-1	-1	1	1	-1	-1	-1	-1	1	1	-1	-1	1	1	1	1	-1	-1;
																															            
            1	-1	-1	1	-1	1	1	-1	-1	1	1	-1	1	-1	-1	1	1	-1	-1	1	-1	1	1	-1	-1	1	1	-1	1	-1	-1	1;
																															            
            1	1	1	1	1	1	1	1	1	1	1	1	1	1	1	1	-1	-1	-1	-1	-1	-1	-1	-1	-1	-1	-1	-1	-1	-1	-1	-1;
																															            
            1	-1	1	-1	1	-1	1	-1	1	-1	1	-1	1	-1	1	-1	-1	1	-1	1	-1	1	-1	1	-1	1	-1	1	-1	1	-1	1;
																															            
            1	1	-1	-1	1	1	-1	-1	1	1	-1	-1	1	1	-1	-1	-1	-1	1	1	-1	-1	1	1	-1	-1	1	1	-1	-1	1	1;
																															            
            1	-1	-1	1	1	-1	-1	1	1	-1	-1	1	1	-1	-1	1	-1	1	1	-1	-1	1	1	-1	-1	1	1	-1	-1	1	1	-1;
																															            
            1	1	1	1	-1	-1	-1	-1	1	1	1	1	-1	-1	-1	-1	-1	-1	-1	-1	1	1	1	1	-1	-1	-1	-1	1	1	1	1;
																															            
            1	-1	1	-1	-1	1	-1	1	1	-1	1	-1	-1	1	-1	1	-1	1	-1	1	1	-1	1	-1	-1	1	-1	1	1	-1	1	-1;
																															            
            1	1	-1	-1	-1	-1	1	1	1	1	-1	-1	-1	-1	1	1	-1	-1	1	1	1	1	-1	-1	-1	-1	1	1	1	1	-1	-1;
																															            
            1	-1	-1	1	-1	1	1	-1	1	-1	-1	1	-1	1	1	-1	-1	1	1	-1	1	-1	-1	1	-1	1	1	-1	1	-1	-1	1;
																															            
            1	1	1	1	1	1	1	1	-1	-1	-1	-1	-1	-1	-1	-1	-1	-1	-1	-1	-1	-1	-1	-1	1	1	1	1	1	1	1	1;
																															            
            1	-1	1	-1	1	-1	1	-1	-1	1	-1	1	-1	1	-1	1	-1	1	-1	1	-1	1	-1	1	1	-1	1	-1	1	-1	1	-1;
																															            
            1	1	-1	-1	1	1	-1	-1	-1	-1	1	1	-1	-1	1	1	-1	-1	1	1	-1	-1	1	1	1	1	-1	-1	1	1	-1	-1;
																															            
            1	-1	-1	1	1	-1	-1	1	-1	1	1	-1	-1	1	1	-1	-1	1	1	-1	-1	1	1	-1	1	-1	-1	1	1	-1	-1	1;
																															            
            1	1	1	1	-1	-1	-1	-1	-1	-1	-1	-1	1	1	1	1	-1	-1	-1	-1	1	1	1	1	1	1	1	1	-1	-1	-1	-1;
																															            
            1	-1	1	-1	-1	1	-1	1	-1	1	-1	1	1	-1	1	-1	-1	1	-1	1	1	-1	1	-1	1	-1	1	-1	-1	1	-1	1;
																															            
            1	1	-1	-1	-1	-1	1	1	-1	-1	1	1	1	1	-1	-1	-1	-1	1	1	1	1	-1	-1	1	1	-1	-1	-1	-1	1	1;
																															            
            1	-1	-1	1	-1	1	1	-1	-1	1	1	-1	1	-1	-1	1	-1	1	1	-1	1	-1	-1	1	1	-1	-1	1	-1	1	1	-1;
        ];

        Increased_Walsh = Walsh(:, repelem(1:size(Walsh, 2), 16));
        
        Ext_Walsh = repmat(Increased_Walsh, [1, 8]);
        
        % 32 streams
        ProcessedInput = reshape(u,4096,32)';
        
        % Polarization
        Polarization = Ext_Walsh;
        assignin('base', "P", Polarization);

y = Polarization;
s = ProcessedInput;

== matlab function E/ DP32 MIMO Demux ==
  data: u input; y1 output; y2 output; y3 output; y4 output; y5 output; y6 output; y7 output; y8 output; y9 output; y10 output; y11 output; y12 output; y13 output; y14 output; y15 output; y16 output; y17 output; y18 output; y19 output; y20 output; y21 output; y22 output; y23 output; y24 output; y25 output; y26 output; y27 output; y28 output; y29 output; y30 output; y31 output; y32 output; c1 parameter; rxDpIndex parameter
function [y1,y2,y3,y4,y5,y6,y7,y8,y9,y10,y11,y12,y13,y14,y15,y16,y17,y18,y19,y20,y21,y22,y23,y24,y25,y26,y27,y28,y29,y30,y31,y32] = fcn(u,c1, rxDpIndex)
    n = 32;
    a = c1;
    r = rxDpIndex;

    Denominator = a*a + a*r*(n-2) - r*r*(n-1);
    S = (1 + r*r*(n-1)/Denominator)/a;
    t = r/Denominator;

    InvHdp = ones(n, n) * t * (-1);
    InvHdp(1:n+1:end) = S;

    TempOutput = u;
    
    for i = 1:4096
        TempOutput(:, i) =  InvHdp * u(:, i);
    end

    y1 = TempOutput(1,:)';
    y2 = TempOutput(2,:)';
    y3 = TempOutput(3,:)';
    y4 = TempOutput(4,:)';
    y5 = TempOutput(5,:)';
    y6 = TempOutput(6,:)';
    y7 = TempOutput(7,:)';
    y8 = TempOutput(8,:)';
    y9 = TempOutput(9,:)';
    y10 = TempOutput(10,:)';
    y11 = TempOutput(11,:)';
    y12 = TempOutput(12,:)';
    y13 = TempOutput(13,:)';
    y14 = TempOutput(14,:)';
    y15 = TempOutput(15,:)';
    y16 = TempOutput(16,:)';
    y17 = TempOutput(17,:)';
    y18 = TempOutput(18,:)';
    y19 = TempOutput(19,:)';
    y20 = TempOutput(20,:)';
    y21 = TempOutput(21,:)';
    y22 = TempOutput(22,:)';
    y23 = TempOutput(23,:)';
    y24 = TempOutput(24,:)';
    y25 = TempOutput(25,:)';
    y26 = TempOutput(26,:)';
    y27 = TempOutput(27,:)';
    y28 = TempOutput(28,:)';
    y29 = TempOutput(29,:)';
    y30 = TempOutput(30,:)';
    y31 = TempOutput(31,:)';
    y32 = TempOutput(32,:)';
